simulink model "Sinwave"  (Simulink 7.8)
settings: Solver=FixedStepDiscrete  StartTime=0.0  StopTime=5  FixedStep=0.0318  RelTol=1e-3
libraries: neural x318
(part 3 of 3)

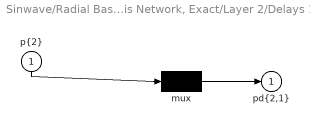
== system Sinwave/Radial Basis Network, Exact/Layer 2/Delays 1 ==
  "p{2}" : Inport  PortDimensions=315
      mask Display: e = 0.06;c1 = [120 230 180]/255;c2 = ([120 230 180]+0)/(256+128);c3 = ([120 230 180]+128)/(256+128);patch([0 1 1 0],[0 0 1 1],c1);patch([0 1 1 1-e 1-e 0+e],[0 0 1 1-e 0+e 0+e],c2);patch([0 0 1 1-e 0+e 0+e],[0 1 1 1-e 1-e 0+e],c3);plot([0 1 1 0 0],[0 0 1 1 0]);
  mux : Mux  Inputs=1
      mask Display: e = 0.06;c1 = [120 150 230]/255;c2 = ([120 150 230]+0)/383;c3 = ([120 150 230]+128)/383;patch([0 1 1 0],[0 0 1 1],c1);patch([0 1 1 1-e 1-e 0+e],[0 0 1 1-e 0+e 0+e],c2);patch([0 0 1 1-e 0+e 0+e],[0 1 1 1-e 1-e 0+e],c3);plot([0 1 1 0 0],[0 0 1 1 0]);disp('Mux')
  "pd{2,1}" : Outport
      mask Display: e = 0.06;c1 = [120 230 180]/255;c2 = ([120 230 180]+0)/(256+128);c3 = ([120 230 180]+128)/(256+128);patch([0 1 1 0],[0 0 1 1],c1);patch([0 1 1 1-e 1-e 0+e],[0 0 1 1-e 0+e 0+e],c2);patch([0 0 1 1-e 0+e 0+e],[0 1 1 1-e 1-e 0+e],c3);plot([0 1 1 0 0],[0 0 1 1 0]);
  wires:
  "p{2}"/1 -> mux/1
  mux/1 -> "pd{2,1}"/1

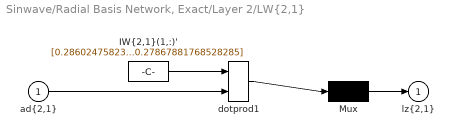
== system Sinwave/Radial Basis Network, Exact/Layer 2/LW{2,1} ==
  "ad{2,1}" : Inport  PortDimensions=315
      mask Display: e = 0.06;c1 = [120 230 180]/255;c2 = ([120 230 180]+0)/(256+128);c3 = ([120 230 180]+128)/(256+128);patch([0 1 1 0],[0 0 1 1],c1);patch([0 1 1 1-e 1-e 0+e],[0 0 1 1-e 0+e 0+e],c2);patch([0 0 1 1-e 0+e 0+e],[0 1 1 1-e 1-e 0+e],c3);plot([0 1 1 0 0],[0 0 1 1 0]);
  "IW{2,1}(1,:)'" : Constant  Value=[0.28602475823221318;1.4875975867205633;-0.48252358032219561;0.070327246551062747;1.5611644816646555;-0.22355991563957986;-0.23593917255130337;1.5591545391524289;0.0838287278473836;-0.48858369753629871;1.4611290033089057;0.41771486168926686;-0.66726717408152314;1.275327093404135;0.75038187220999919;-0.7571634331419721;1.0171617115944529;1.0542329915068223;-0.75081501953378027;0.70804933714537244;1.3040618174073286;-0.64874857484742254;0.37363282661120023;1.4791434444136404;-0.45943116613724039;0.041654177152025282;1.5649537271974954;-0.19856788824555074;-0.26034685030419052;1.554374151731295;0.11220097467157845;-0.50731733108979815;1.448282361741607;0.4470951496883756;-0.67876947778781116;1.2554793525258814;0.77833301430843371;-0.76048023376991569;0.99195937187279282;1.078436260463475;-0.74567116708374037;0.67958309449365062;1.3225093966322885;-0.63557078491422947;0.3442641386666897;1.4903049887405007;-0.43931262102316398;0.013819365184402469;1.5679033148452701;-0.17317755046841979;-0.28433870988797733;1.5488670954624317;0.1407568135373144;-0.5254759594624302;1.4347755072397665;0.47644759942419795;-0.68958850011168582;1.2350931801125302;0.80604710070834096;-0.76306214266386885;0.96638504546890158;1.1022129220816703;-0.7398017766241024;0.65094216871188182;1.3403762066946865;-0.62173699873265065;0.3149325622316641;1.5007797806123551;-0.41866204052349942;-0.013769619272249249;1.5701171372720697;-0.14742327392039065;-0.30789641893008451;1.5426362976568053;0.16947830350094706;-0.54304812983812889;1.4206169738936383;0.50575367076251321;-0.69971740744046984;1.2141814524925751;0.83350662660129671;-0.76490752903530479;0.94045488567557434;1.1255479585123143;-0.73321055538768909;0.62214465002266806;1.3576509625342839;-0.60725595401852384;0.28565662375841289;1.5105612039261653;-0.39749246798745608;-0.041095350424057507;1.5715937961802335;-0.12132132555459978;-0.33100509787651328;1.5356856938198435;0.19834730345374652;-0.56002274325746071;1.405815704536344;0.53499485336058272;-0.7091498021391619;1.1927573779613894;0.86069424796220428;-0.7660152272986297;0.91418527053756016;1.1484266308462392;-0.72590166653109167;0.59320872755597664;1.374322753045099;-0.59213679731008451;0.25645481455724251;1.5196430805253065;-0.37581727457084307;-0.068140568753499386;1.5723323588803324;-0.094888191921072104;-0.35365015079036777;1.5280196741018859;0.22734557911667369;-0.57638907819073426;1.3903810479668612;0.56415267786069112;-0.71787972650515408;1.1708344884236619;0.88759279250671264;-0.76638453780789195;0.88759279250672596;1.170834488423641;-0.71787972650517162;0.56415267786070267;1.3903810479668679;-0.57638907819076357;0.22734557911670825;1.5280196741018794;-0.35365015079034995;-0.094888191921049359;1.5723323588803377;-0.068140568753528835;-0.37581727457083136;1.5196430805253169;0.25645481455720315;-0.59213679731008206;1.3743227530450914;0.59320872755597465;-0.72590166653108201;1.1484266308462661;0.91418527053750709;-0.76601522729862381;0.86069424796218008;1.1927573779614074;-0.70914980213916967;0.53499485336059516;1.4058157045363446;-0.56002274325747514;0.19834730345380858;1.5356856938198178;-0.33100509787648902;-0.12132132555460536;1.5715937961802404;-0.041095350424082522;-0.39749246798745114;1.5105612039261775;0.28565662375837536;-0.60725595401852006;1.3576509625342914;0.62214465002263175;-0.73321055538767732;1.1255479585123409;0.94045488567555657;-0.76490752903530723;0.83350662660132191;1.2141814524925756;-0.69971740744045996;0.50575367076254418;1.4206169738936298;-0.54304812983815209;0.16947830350098303;1.5426362976567967;-0.30789641893010694;-0.14742327392041307;1.5701171372720795;-0.013769619272267601;-0.41866204052346773;1.5007797806123739;0.31493256223158778;-0.62173699873260613;1.3403762066946583;0.65094216871189181;-0.73980177662409363;1.1022129220817045;0.96638504546886528;-0.76306214266387506;0.80604710070837804;1.2350931801124927;-0.68958850011167305;0.4764475994242075;1.4347755072397592;-0.52547595946245684;0.14075681353735348 ...(+2300 chars)]
      mask Display: e = 0.06;c1 = [120 150 230]/255;c2 = ([120 150 230]+0)/383;c3 = ([120 150 230]+128)/383;patch([0 1 1 0],[0 0 1 1],c1);patch([0 1 1 1-e 1-e 0+e],[0 0 1 1-e 0+e 0+e],c2);patch([0 0 1 1-e 0+e 0+e],[0 1 1 1-e 1-e 0+e],c3);plot([0 1 1 0 0],[0 0 1 1 0]);disp('weights');
  Mux : Mux  Inputs=1
      mask Display: e = 0.06;c1 = [120 150 230]/255;c2 = ([120 150 230]+0)/383;c3 = ([120 150 230]+128)/383;patch([0 1 1 0],[0 0 1 1],c1);patch([0 1 1 1-e 1-e 0+e],[0 0 1 1-e 0+e 0+e],c2);patch([0 0 1 1-e 0+e 0+e],[0 1 1 1-e 1-e 0+e],c3);plot([0 1 1 0 0],[0 0 1 1 0]);disp('Mux');
  dotprod1 : neural/Weight Functions/dotprod
  "lz{2,1}" : Outport
      mask Display: e = 0.06;c1 = [120 230 180]/255;c2 = ([120 230 180]+0)/(256+128);c3 = ([120 230 180]+128)/(256+128);patch([0 1 1 0],[0 0 1 1],c1);patch([0 1 1 1-e 1-e 0+e],[0 0 1 1-e 0+e 0+e],c2);patch([0 0 1 1-e 0+e 0+e],[0 1 1 1-e 1-e 0+e],c3);plot([0 1 1 0 0],[0 0 1 1 0]);
  wires:
  "IW{2,1}(1,:)'"/1 -> dotprod1/1
  "ad{2,1}"/1 -> dotprod1/2
  dotprod1/1 -> Mux/1
  Mux/1 -> "lz{2,1}"/1
